simulink model "processor_ks"  (R2025a)
settings: Solver=VariableStepAuto  StartTime=0.0  StopTime=10.0  RelTol=1e-3
(part 1 of 2)
settings Model: Creator=Krutyanjay  LastModifiedBy=Krutyanjay

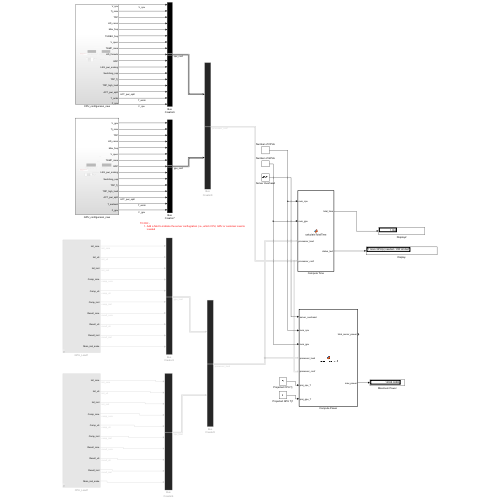
[thumbnail: Simulink's stored preview of the top-level diagram]
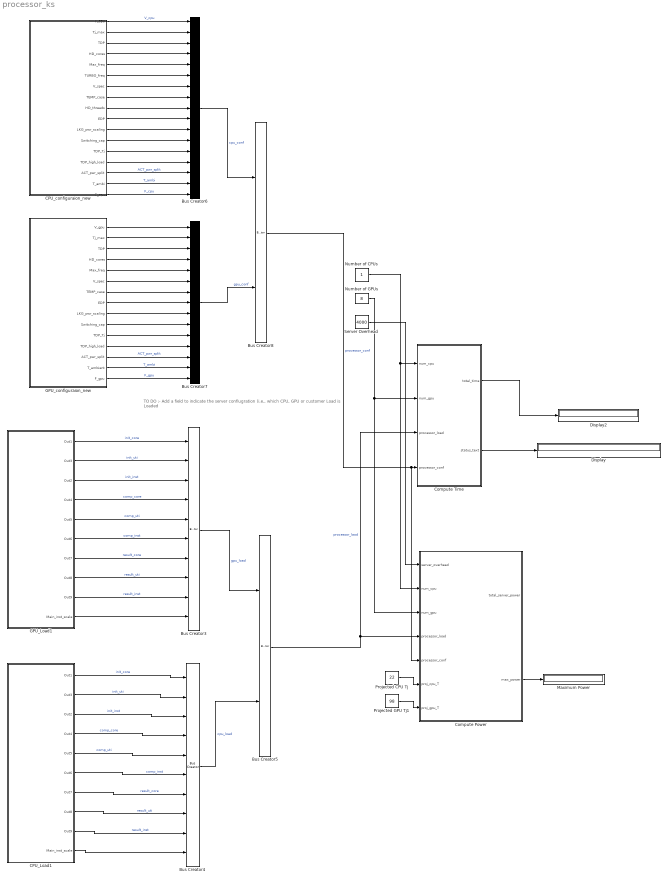
== system processor_ks ==
  note: TO DO :-
      | Add a field to indicate the server confiugration (i.e., which CPU, GPU or customer Load is Loaded
  Bus Creator3 : BusCreator  Inputs=10  OutDataTypeStr=Bus: gpu_load
  Bus Creator4 : BusCreator  Inputs=10  OutDataTypeStr=Bus: cpu_load
  Bus Creator5 : BusCreator  Inputs=2  OutDataTypeStr=Bus: processor_load
  Bus Creator6 : BusCreator  Inputs=17  OutDataTypeStr=Bus: cpu_conf
  Bus Creator7 : BusCreator  Inputs=15  OutDataTypeStr=Bus: gpu_conf
  Bus Creator8 : BusCreator  Inputs=2  OutDataTypeStr=Bus: processor_conf
  CPU_Load1 : Subsystem  mask{Init_core=30, Init_uti=0.5, Init_inst=500000, Comp_core=0, Comp_uti=0, Comp_inst=0, Result_core=20, Result_uti=0.5, Result_inst=100000, Main_inst_scale=1}
      mask prompts: Init_core "Initilization Phase cores"; Init_uti "Total initilization core utilization"; Init_inst "Number of instructions for initilization"; Comp_core "Compute Phase cores"; Comp_uti "Total Compute core utilization"; Comp_inst "Number of isntrutction for compute"; Result_core "Result Phase cores"; Result_uti "Total result core utilization"; Result_inst "Number of instructions for result"; Main_inst_scale "Main Phase Instruction scaling"
      mask DialogControl saveButton Prompt: Save to CSV
      mask DialogControl loadButton Prompt: Load from CSV
  CPU_configuraion_new : Subsystem
  Compute Power : MATLAB Function  TreatAsAtomicUnit=on
  Compute Time : MATLAB Function  TreatAsAtomicUnit=on
  Display : Display
  Display2 : Display
  GPU_Load1 : Subsystem  mask{Init_core=12, Init_uti=0.1, Init_inst=40000, Comp_core=250000, Comp_uti=0.75, Comp_inst=1000000000000000, Result_core=5, Result_uti=0.1, Result_inst=10000, Main_inst_scale=2.8}
      mask prompts: Init_core "Initilization Phase cores"; Init_uti "Total initilization core utilization"; Init_inst "Number of instructions for initilization"; Comp_core "Compute Phase cores"; Comp_uti "Total Compute core utilization"; Comp_inst "Number of isntrutction for compute"; Result_core "Result Phase cores"; Result_uti "Total result core utilization"; Result_inst "Number of instructions for result"; Main_inst_scale "Main Phase Instruction Scaling"
      mask DialogControl saveButton Prompt: Save to CSV
      mask DialogControl loadButton Prompt: Load from CSV
  GPU_configuraion_new : Subsystem
  Maximum Power : Display
  Number of CPUs : Constant
  Number of GPUs : Constant  Value=8
  Projected CPU Tj : Constant  Value=22
  Projected GPU Tj1 : Constant  Value=98
  Server Overhead : Constant  Value=4000
  wires:
  GPU_Load1/7(Out7) -> Bus Creator3/7  "result_core"
  CPU_Load1/5(Out5) -> Bus Creator4/5  "comp_uti"
  GPU_Load1/2(Out3) -> Bus Creator3/2  "init_uti"
  GPU_Load1/3(Out2) -> Bus Creator3/3  "init_inst"
  CPU_Load1/8(Out8) -> Bus Creator4/8  "result_uti"
  CPU_Load1/1(Out1) -> Bus Creator4/1  "init_core"
  CPU_Load1/3(Out2) -> Bus Creator4/3  "init_inst"
  GPU_Load1/6(Out6) -> Bus Creator3/6  "comp_inst"
  GPU_Load1/1(Out1) -> Bus Creator3/1  "init_core"
  CPU_Load1/4(Out4) -> Bus Creator4/4  "comp_core"
  GPU_Load1/4(Out4) -> Bus Creator3/4  "comp_core"
  GPU_Load1/9(Out9) -> Bus Creator3/9  "result_inst"
  CPU_Load1/2(Out3) -> Bus Creator4/2  "init_uti"
  CPU_Load1/9(Out9) -> Bus Creator4/9  "result_inst"
  GPU_Load1/8(Out8) -> Bus Creator3/8  "result_uti"
  CPU_Load1/6(Out6) -> Bus Creator4/6  "comp_inst"
  GPU_Load1/5(Out5) -> Bus Creator3/5  "comp_uti"
  CPU_Load1/7(Out7) -> Bus Creator4/7  "result_core"
  Bus Creator6/1 -> Bus Creator8/1  "cpu_conf"
  Bus Creator7/1 -> Bus Creator8/2  "gpu_conf"
  Bus Creator8/1 -> Compute Power/5(processor_conf), Compute Time/4(processor_conf)  "processor_conf"
  Bus Creator5/1 -> Compute Time/3(processor_load), Compute Power/4(processor_load)  "processor_laod"
  Compute Time/1(total_time) -> Display2/1
  Number of CPUs/1 -> Compute Time/1(num_cpu), Compute Power/2(num_cpu)
  Number of GPUs/1 -> Compute Power/3(num_gpu), Compute Time/2(num_gpu)
  Server Overhead/1 -> Compute Power/1(server_overhead)
  Compute Power/2(max_power) -> Maximum Power/1
  Compute Time/2(status_text) -> Display/1
  GPU_configuraion_new/1(V_gpu) -> Bus Creator7/1
  GPU_configuraion_new/2(Tj_max) -> Bus Creator7/2
  GPU_configuraion_new/3(TDP) -> Bus Creator7/3
  GPU_configuraion_new/4(HD_cores) -> Bus Creator7/4
  GPU_configuraion_new/5(Max_freq) -> Bus Creator7/5
  GPU_configuraion_new/6(V_spec) -> Bus Creator7/6
  GPU_configuraion_new/7(TEMP_case) -> Bus Creator7/7
  GPU_configuraion_new/8(EDP) -> Bus Creator7/8
  GPU_configuraion_new/9(LKG_pwr_scaling) -> Bus Creator7/9
  GPU_configuraion_new/10(Switching_cap) -> Bus Creator7/10
  GPU_configuraion_new/11(TDP_Tj) -> Bus Creator7/11
  GPU_configuraion_new/12(TDP_high_load) -> Bus Creator7/12
  GPU_configuraion_new/13(ACT_pwr_split) -> Bus Creator7/13  "ACT_pwr_split"
  CPU_configuraion_new/1(V_cpu) -> Bus Creator6/1  "V_cpu"
  CPU_configuraion_new/2(Tj_max) -> Bus Creator6/2
  CPU_configuraion_new/3(TDP) -> Bus Creator6/3
  CPU_configuraion_new/4(HD_cores) -> Bus Creator6/4
  CPU_configuraion_new/5(Max_freq) -> Bus Creator6/5
  CPU_configuraion_new/6(TURBO_freq) -> Bus Creator6/6
  CPU_configuraion_new/7(V_spec) -> Bus Creator6/7
  CPU_configuraion_new/8(TEMP_case) -> Bus Creator6/8
  CPU_configuraion_new/9(HD_threads) -> Bus Creator6/9
  CPU_configuraion_new/10(EDP) -> Bus Creator6/10
  CPU_configuraion_new/11(LKG_pwr_scaling) -> Bus Creator6/11
  CPU_configuraion_new/12(Switching_cap) -> Bus Creator6/12
  CPU_configuraion_new/13(TDP_Tj) -> Bus Creator6/13
  CPU_configuraion_new/14(TDP_high_load) -> Bus Creator6/14
  CPU_configuraion_new/15(ACT_pwr_split) -> Bus Creator6/15  "ACT_pwr_split"
  Bus Creator3/1 -> Bus Creator5/1  "gpu_load"
  Bus Creator4/1 -> Bus Creator5/2  "cpu_load"
  CPU_configuraion_new/16(T_ambi) -> Bus Creator6/16  "T_ambi"
  GPU_configuraion_new/14(T_ambient) -> Bus Creator7/14  "T_ambi"
  CPU_configuraion_new/17(F_cpu) -> Bus Creator6/17  "F_cpu"
  GPU_configuraion_new/15(F_gpu) -> Bus Creator7/15  "F_gpu"
  GPU_Load1/10(Main_inst_scale) -> Bus Creator3/10
  CPU_Load1/10(Main_inst_scale) -> Bus Creator4/10
  Projected CPU Tj/1 -> Compute Power/6(proj_cpu_T)
  Projected GPU Tj1/1 -> Compute Power/7(proj_gpu_T)

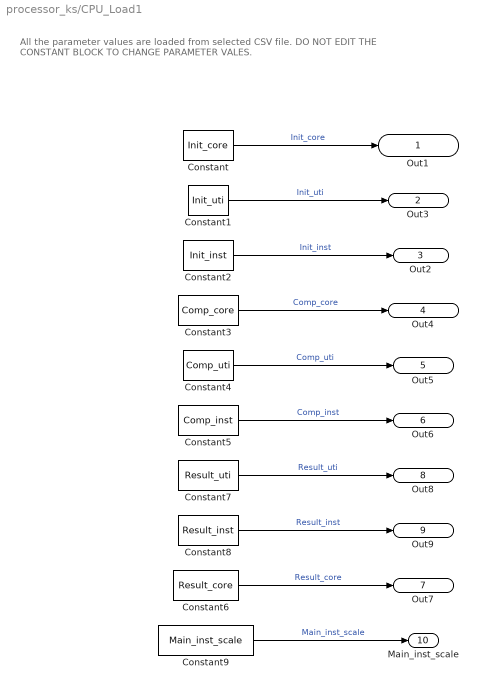
== system processor_ks/CPU_Load1 ==
  note: All the parameter values are loaded from selected CSV file.
      | DO NOT EDIT THE CONSTANT BLOCK TO CHANGE PARAMETER VALES.
  Constant : Constant  Value=Init_core
  Constant1 : Constant  Value=Init_uti
  Constant2 : Constant  Value=Init_inst
  Constant3 : Constant  Value=Comp_core
  Constant4 : Constant  Value=Comp_uti
  Constant5 : Constant  Value=Comp_inst
  Constant6 : Constant  Value=Result_core
  Constant7 : Constant  Value=Result_uti
  Constant8 : Constant  Value=Result_inst
  Constant9 : Constant  Value=Main_inst_scale
  Out1 : Outport
  Out3 : Outport  Port=2
  Out2 : Outport  Port=3
  Out4 : Outport  Port=4
  Out5 : Outport  Port=5
  Out6 : Outport  Port=6
  Out7 : Outport  Port=7
  Out8 : Outport  Port=8
  Out9 : Outport  Port=9
  Main_inst_scale : Outport  Port=10
  wires:
  Constant7/1 -> Out8/1  "Result_uti"
  Constant5/1 -> Out6/1  "Comp_inst"
  Constant3/1 -> Out4/1  "Comp_core"
  Constant1/1 -> Out3/1  "Init_uti"
  Constant4/1 -> Out5/1  "Comp_uti"
  Constant6/1 -> Out7/1  "Result_core"
  Constant/1 -> Out1/1  "Init_core"
  Constant2/1 -> Out2/1  "Init_inst"
  Constant8/1 -> Out9/1  "Result_inst"
  Constant9/1 -> Main_inst_scale/1  "Main_inst_scale"

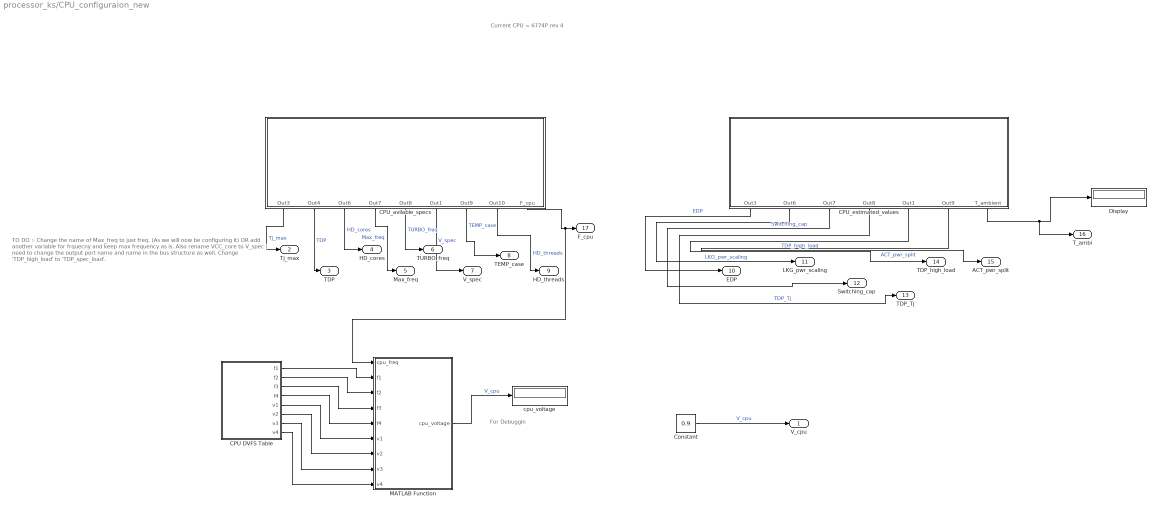
== system processor_ks/CPU_configuraion_new ==
  note: TO DO :-
      | Change the name of Max_freq to just freq. (As we will now be configuring it)
      | OR add another variable for frquecny and keep max frequency as is.
      | Also rename VCC_core to V_spec ( need to change the output port name and name in the bus structure as well.
      | Change 'TDP_high_load' to 'TDP_spec_load'.
  note: For Debuggin
  note: Current CPU = 6774P rev 4
  CPU DVFS Table : Subsystem  mask{F1=2.5e9, F2=2.3e9, F3=1.8e9, F4=1.4e9, V1=1.5, V2=1.3, V3=1.1, V4=0.9, loaded_device_name=hello}
      mask prompts: loaded_device_name "Device DVFS"
      mask DialogControl save_dvfs_button Prompt: Save To CSV
      mask DialogControl load_dvfs_button Prompt: Load From CSV
  CPU_avilable_specs : Subsystem  mask{TURBO_freq=3.9e9, V_spec=1.5, TEMP_case=85, Tj_max=100, HD_cores=40, Max_freq=2500000000, TDP=235, HD_threads=128, F_cpu=1.4e9}
      mask DialogControl save_button Prompt: Save To CSV
      mask DialogControl load_button Prompt: Load From CSV
  CPU_estimated_values : Subsystem  mask{EDP=587.5, LKG_pwr_scaling=394.5, Switching_cap=28.35, TDP_Tj=70, TDP_high_load=0.7, ACT_pwr_split=0.5, T_ambient=20}
      mask DialogControl save_button Prompt: Save To CSV
      mask DialogControl load_button Prompt: Load From CSV
  Constant : Constant  Value=0.9
  Display : Display
  MATLAB Function : MATLAB Function  TreatAsAtomicUnit=on
  cpu_voltage : Display
  V_cpu : Outport
  Tj_max : Outport  Port=2
  TDP : Outport  Port=3
  HD_cores : Outport  Port=4
  Max_freq : Outport  Port=5
  TURBO_freq : Outport  Port=6
  V_spec : Outport  Port=7
  TEMP_case : Outport  Port=8
  HD_threads : Outport  Port=9
  EDP : Outport  Port=10
  LKG_pwr_scaling : Outport  Port=11
  Switching_cap : Outport  Port=12
  TDP_Tj : Outport  Port=13
  TDP_high_load : Outport  Port=14
  ACT_pwr_split : Outport  Port=15
  T_ambi : Outport  Port=16
  F_cpu : Outport  Port=17
  wires:
  CPU_avilable_specs/1(Out3) -> Tj_max/1  "Tj_max"
  CPU_avilable_specs/2(Out4) -> TDP/1  "TDP"
  CPU_avilable_specs/3(Out6) -> HD_cores/1  "HD_cores"
  CPU_avilable_specs/4(Out7) -> Max_freq/1  "Max_freq"
  CPU_avilable_specs/5(Out8) -> TURBO_freq/1  "TURBO_freq"
  CPU_avilable_specs/7(Out9) -> TEMP_case/1  "TEMP_case"
  CPU_avilable_specs/8(Out10) -> HD_threads/1  "HD_threads"
  CPU_estimated_values/1(Out3) -> EDP/1  "EDP"
  CPU_estimated_values/2(Out6) -> LKG_pwr_scaling/1  "LKG_pwr_scaling"
  CPU_estimated_values/3(Out7) -> Switching_cap/1  "Switching_cap"
  CPU_estimated_values/4(Out8) -> TDP_Tj/1  "TDP_Tj"
  CPU_estimated_values/5(Out1) -> TDP_high_load/1  "TDP_high_load"
  CPU_estimated_values/6(Out9) -> ACT_pwr_split/1  "ACT_pwr_split"
  CPU DVFS Table/1(f1) -> MATLAB Function/2(f1)
  CPU DVFS Table/2(f2) -> MATLAB Function/3(f2)
  CPU DVFS Table/3(f3) -> MATLAB Function/4(f3)
  CPU DVFS Table/4(f4) -> MATLAB Function/5(f4)
  CPU DVFS Table/5(v1) -> MATLAB Function/6(v1)
  CPU DVFS Table/6(v2) -> MATLAB Function/7(v2)
  CPU DVFS Table/7(v3) -> MATLAB Function/8(v3)
  CPU DVFS Table/8(v4) -> MATLAB Function/9(v4)
  MATLAB Function/1(cpu_voltage) -> cpu_voltage/1  "V_cpu"
  CPU_avilable_specs/6(Out1) -> V_spec/1  "V_spec"
  CPU_estimated_values/7(T_ambient) -> T_ambi/1, Display/1
  CPU_avilable_specs/9(F_cpu) -> MATLAB Function/1(cpu_freq), F_cpu/1
  Constant/1 -> V_cpu/1  "V_cpu"

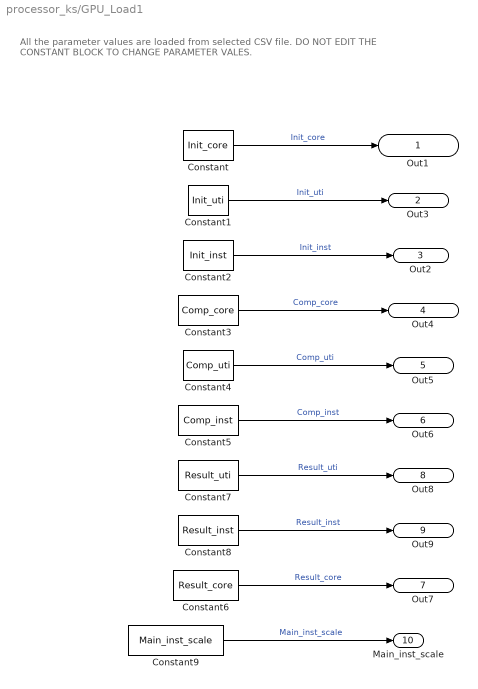
== system processor_ks/GPU_Load1 ==
  note: All the parameter values are loaded from selected CSV file.
      | DO NOT EDIT THE CONSTANT BLOCK TO CHANGE PARAMETER VALES.
  Constant : Constant  Value=Init_core
  Constant1 : Constant  Value=Init_uti
  Constant2 : Constant  Value=Init_inst
  Constant3 : Constant  Value=Comp_core
  Constant4 : Constant  Value=Comp_uti
  Constant5 : Constant  Value=Comp_inst
  Constant6 : Constant  Value=Result_core
  Constant7 : Constant  Value=Result_uti
  Constant8 : Constant  Value=Result_inst
  Constant9 : Constant  Value=Main_inst_scale
  Out1 : Outport
  Out3 : Outport  Port=2
  Out2 : Outport  Port=3
  Out4 : Outport  Port=4
  Out5 : Outport  Port=5
  Out6 : Outport  Port=6
  Out7 : Outport  Port=7
  Out8 : Outport  Port=8
  Out9 : Outport  Port=9
  Main_inst_scale : Outport  Port=10
  wires:
  Constant7/1 -> Out8/1  "Result_uti"
  Constant5/1 -> Out6/1  "Comp_inst"
  Constant3/1 -> Out4/1  "Comp_core"
  Constant1/1 -> Out3/1  "Init_uti"
  Constant4/1 -> Out5/1  "Comp_uti"
  Constant6/1 -> Out7/1  "Result_core"
  Constant/1 -> Out1/1  "Init_core"
  Constant2/1 -> Out2/1  "Init_inst"
  Constant8/1 -> Out9/1  "Result_inst"
  Constant9/1 -> Main_inst_scale/1  "Main_inst_scale"

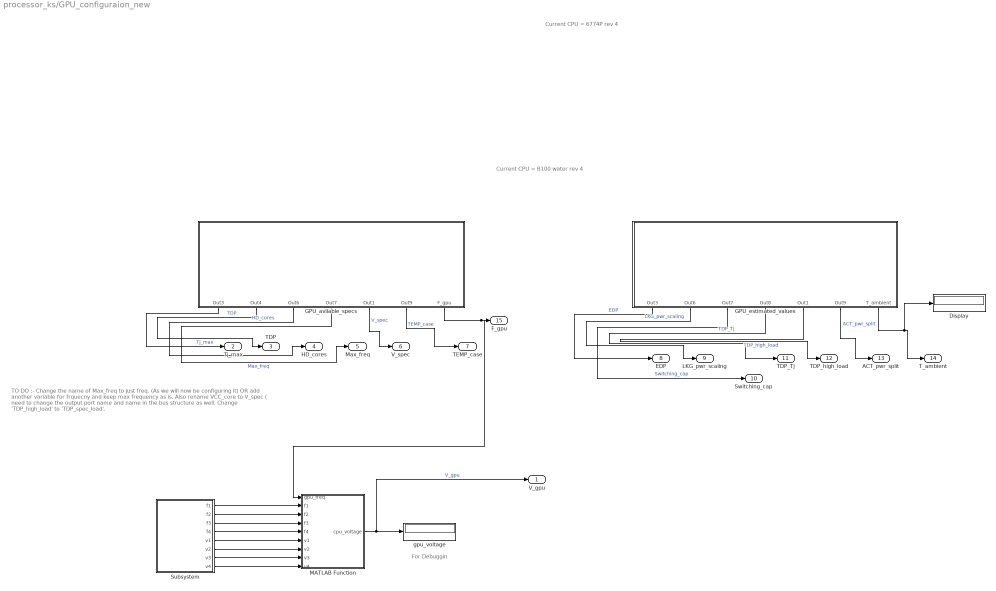
== system processor_ks/GPU_configuraion_new ==
  note: For Debuggin
  note: TO DO :-
      | Change the name of Max_freq to just freq. (As we will now be configuring it)
      | OR add another variable for frquecny and keep max frequency as is.
      | Also rename VCC_core to V_spec ( need to change the output port name and name in the bus structure as well.
      | Change 'TDP_high_load' to 'TDP_spec_load'.
  note: Current CPU = 6774P rev 4
  note: Current CPU = B100 water rev 4
  Display : Display
  GPU_avilable_specs : Subsystem  mask{V_spec=1, TEMP_case=85, Tj_max=95, HD_cores=30000, Max_freq=1900000000, TDP=1400, F_gpu=1.4e9}
      mask DialogControl save_button Prompt: Save To CSV
      mask DialogControl load_button Prompt: Load From CSV
  GPU_estimated_values : Subsystem  mask{EDP=2286.7, LKG_pwr_scaling=1, Switching_cap=368.42, TDP_Tj=70, TDP_high_load=0.75, ACT_pwr_split=0.5, T_ambient=20}
      mask DialogControl save_button Prompt: Save To CSV
      mask DialogControl load_button Prompt: Load From CSV
  MATLAB Function : MATLAB Function  TreatAsAtomicUnit=on
  Subsystem : Subsystem  mask{F1=1.9e9, F2=1.7e9, F3=1.4e9, F4=1.3e9, V1=1, V2=0.8, V3=0.7, V4=0.5, loaded_device_name=0}
      mask prompts: loaded_device_name "Device's DVFS"
      mask DialogControl save_dvfs_button Prompt: Save To CSV
      mask DialogControl load_dvfs_button Prompt: Load from CSV
  gpu_voltage : Display
  V_gpu : Outport
  Tj_max : Outport  Port=2
  TDP : Outport  Port=3
  HD_cores : Outport  Port=4
  Max_freq : Outport  Port=5
  V_spec : Outport  Port=6
  TEMP_case : Outport  Port=7
  EDP : Outport  Port=8
  LKG_pwr_scaling : Outport  Port=9
  Switching_cap : Outport  Port=10
  TDP_Tj : Outport  Port=11
  TDP_high_load : Outport  Port=12
  ACT_pwr_split : Outport  Port=13
  T_ambient : Outport  Port=14
  F_gpu : Outport  Port=15
  wires:
  GPU_avilable_specs/1(Out3) -> Tj_max/1  "Tj_max"
  GPU_avilable_specs/2(Out4) -> TDP/1  "TDP"
  GPU_avilable_specs/3(Out6) -> HD_cores/1  "HD_cores"
  GPU_avilable_specs/4(Out7) -> Max_freq/1  "Max_freq"
  GPU_avilable_specs/5(Out1) -> V_spec/1  "V_spec"
  GPU_avilable_specs/6(Out9) -> TEMP_case/1  "TEMP_case"
  GPU_estimated_values/1(Out3) -> EDP/1  "EDP"
  GPU_estimated_values/2(Out6) -> LKG_pwr_scaling/1  "LKG_pwr_scaling"
  GPU_estimated_values/3(Out7) -> Switching_cap/1  "Switching_cap"
  GPU_estimated_values/4(Out8) -> TDP_Tj/1  "TDP_Tj"
  GPU_estimated_values/5(Out1) -> TDP_high_load/1  "TDP_high_load"
  GPU_estimated_values/6(Out9) -> ACT_pwr_split/1  "ACT_pwr_split"
  MATLAB Function/1(cpu_voltage) -> V_gpu/1, gpu_voltage/1  "V_gpu"
  Subsystem/3(f3) -> MATLAB Function/4(f3)
  Subsystem/2(f2) -> MATLAB Function/3(f2)
  Subsystem/6(v2) -> MATLAB Function/7(v2)
  Subsystem/8(v4) -> MATLAB Function/9(v4)
  Subsystem/7(v3) -> MATLAB Function/8(v3)
  Subsystem/1(f1) -> MATLAB Function/2(f1)
  Subsystem/4(f4) -> MATLAB Function/5(f4)
  Subsystem/5(v1) -> MATLAB Function/6(v1)
  GPU_estimated_values/7(T_ambient) -> Display/1, T_ambient/1
  GPU_avilable_specs/7(F_gpu) -> MATLAB Function/1(gpu_freq), F_gpu/1

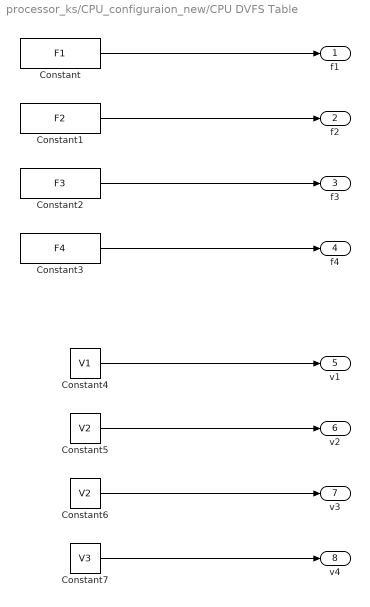
== system processor_ks/CPU_configuraion_new/CPU DVFS Table ==
  Constant : Constant  Value=F1
  Constant1 : Constant  Value=F2
  Constant2 : Constant  Value=F3
  Constant3 : Constant  Value=F4
  Constant4 : Constant  Value=V1
  Constant5 : Constant  Value=V2
  Constant6 : Constant  Value=V2
  Constant7 : Constant  Value=V3
  f1 : Outport
  f2 : Outport  Port=2
  f3 : Outport  Port=3
  f4 : Outport  Port=4
  v1 : Outport  Port=5
  v2 : Outport  Port=6
  v3 : Outport  Port=7
  v4 : Outport  Port=8
  wires:
  Constant/1 -> f1/1
  Constant1/1 -> f2/1
  Constant2/1 -> f3/1
  Constant3/1 -> f4/1
  Constant7/1 -> v4/1
  Constant6/1 -> v3/1
  Constant5/1 -> v2/1
  Constant4/1 -> v1/1

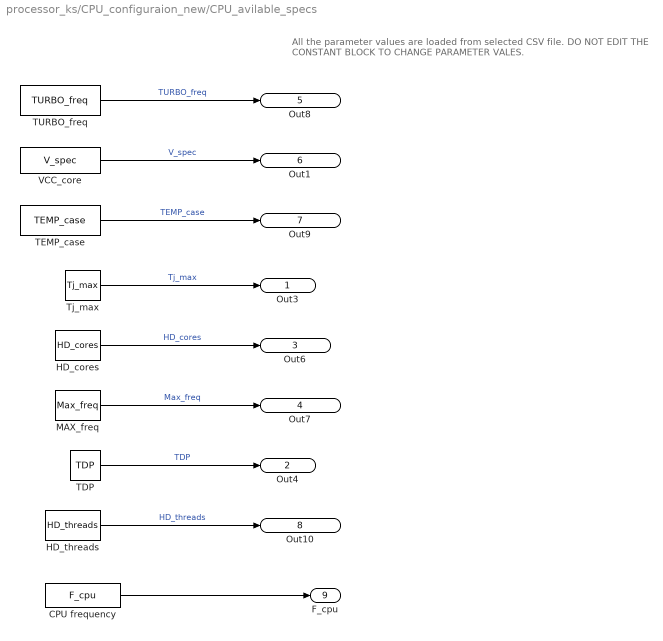
== system processor_ks/CPU_configuraion_new/CPU_avilable_specs ==
  note: All the parameter values are loaded from selected CSV file.
      | DO NOT EDIT THE CONSTANT BLOCK TO CHANGE PARAMETER VALES.
  CPU frequency : Constant  Value=F_cpu
  HD_cores : Constant  Value=HD_cores
  HD_threads : Constant  Value=HD_threads
  MAX_freq : Constant  Value=Max_freq
  TDP : Constant  Value=TDP
  TEMP_case : Constant  Value=TEMP_case
  TURBO_freq : Constant  Value=TURBO_freq
  Tj_max : Constant  Value=Tj_max
  VCC_core : Constant  Value=V_spec
  Out3 : Outport
  Out4 : Outport  Port=2
  Out6 : Outport  Port=3
  Out7 : Outport  Port=4
  Out8 : Outport  Port=5
  Out1 : Outport  Port=6
  Out9 : Outport  Port=7
  Out10 : Outport  Port=8
  F_cpu : Outport  Port=9
  wires:
  HD_threads/1 -> Out10/1  "HD_threads"
  TDP/1 -> Out4/1  "TDP"
  MAX_freq/1 -> Out7/1  "Max_freq"
  HD_cores/1 -> Out6/1  "HD_cores"
  Tj_max/1 -> Out3/1  "Tj_max"
  TEMP_case/1 -> Out9/1  "TEMP_case"
  TURBO_freq/1 -> Out8/1  "TURBO_freq"
  VCC_core/1 -> Out1/1  "V_spec"
  CPU frequency/1 -> F_cpu/1

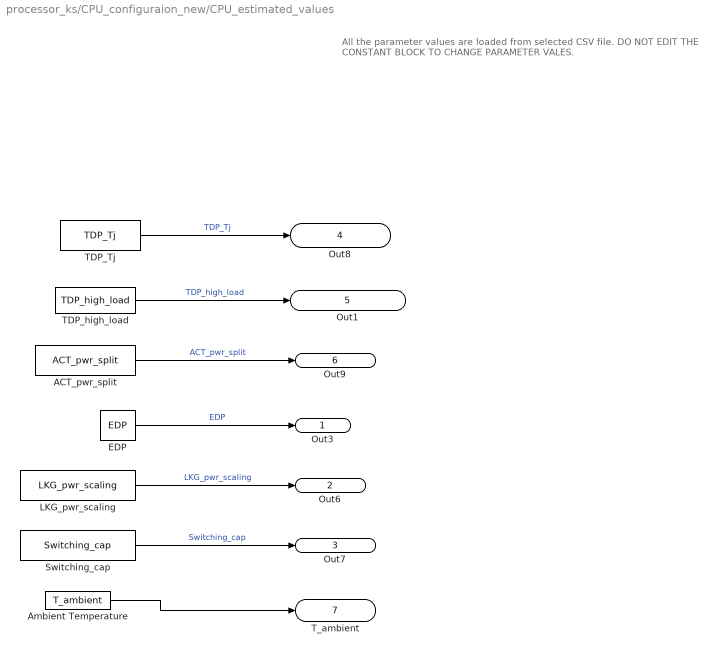
== system processor_ks/CPU_configuraion_new/CPU_estimated_values ==
  note: All the parameter values are loaded from selected CSV file.
      | DO NOT EDIT THE CONSTANT BLOCK TO CHANGE PARAMETER VALES.
  ACT_pwr_split : Constant  Value=ACT_pwr_split
  Ambient Temperature : Constant  Value=T_ambient
  EDP : Constant  Value=EDP
  LKG_pwr_scaling : Constant  Value=LKG_pwr_scaling
  Switching_cap : Constant  Value=Switching_cap
  TDP_Tj : Constant  Value=TDP_Tj
  TDP_high_load : Constant  Value=TDP_high_load
  Out3 : Outport
  Out6 : Outport  Port=2
  Out7 : Outport  Port=3
  Out8 : Outport  Port=4
  Out1 : Outport  Port=5
  Out9 : Outport  Port=6
  T_ambient : Outport  Port=7
  wires:
  Switching_cap/1 -> Out7/1  "Switching_cap"
  LKG_pwr_scaling/1 -> Out6/1  "LKG_pwr_scaling"
  EDP/1 -> Out3/1  "EDP"
  ACT_pwr_split/1 -> Out9/1  "ACT_pwr_split"
  TDP_Tj/1 -> Out8/1  "TDP_Tj"
  TDP_high_load/1 -> Out1/1  "TDP_high_load"
  Ambient Temperature/1 -> T_ambient/1

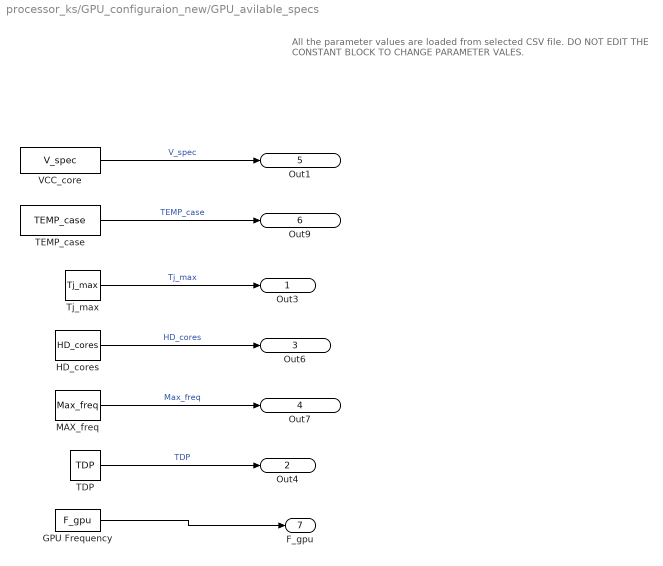
== system processor_ks/GPU_configuraion_new/GPU_avilable_specs ==
  note: All the parameter values are loaded from selected CSV file.
      | DO NOT EDIT THE CONSTANT BLOCK TO CHANGE PARAMETER VALES.
  GPU Frequency : Constant  Value=F_gpu
  HD_cores : Constant  Value=HD_cores
  MAX_freq : Constant  Value=Max_freq
  TDP : Constant  Value=TDP
  TEMP_case : Constant  Value=TEMP_case
  Tj_max : Constant  Value=Tj_max
  VCC_core : Constant  Value=V_spec
  Out3 : Outport
  Out4 : Outport  Port=2
  Out6 : Outport  Port=3
  Out7 : Outport  Port=4
  Out1 : Outport  Port=5
  Out9 : Outport  Port=6
  F_gpu : Outport  Port=7
  wires:
  TDP/1 -> Out4/1  "TDP"
  MAX_freq/1 -> Out7/1  "Max_freq"
  HD_cores/1 -> Out6/1  "HD_cores"
  Tj_max/1 -> Out3/1  "Tj_max"
  TEMP_case/1 -> Out9/1  "TEMP_case"
  VCC_core/1 -> Out1/1  "V_spec"
  GPU Frequency/1 -> F_gpu/1

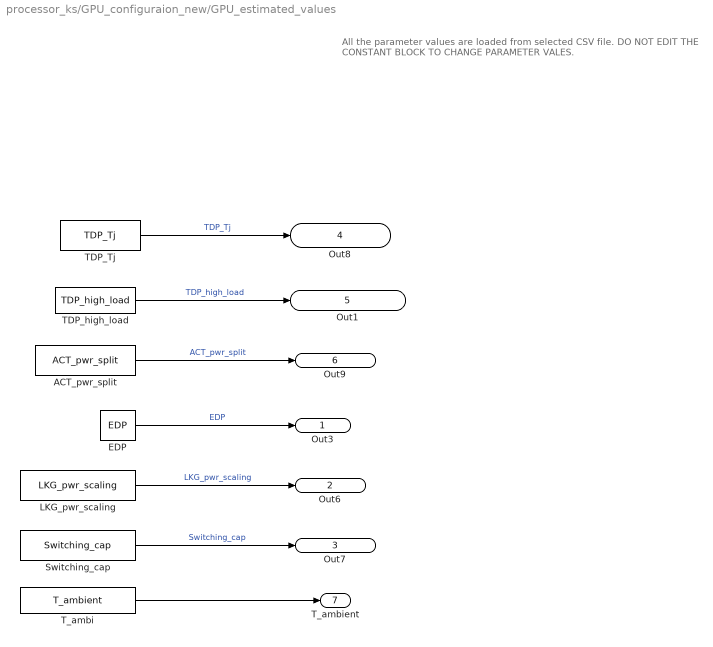
== system processor_ks/GPU_configuraion_new/GPU_estimated_values ==
  note: All the parameter values are loaded from selected CSV file.
      | DO NOT EDIT THE CONSTANT BLOCK TO CHANGE PARAMETER VALES.
  ACT_pwr_split : Constant  Value=ACT_pwr_split
  EDP : Constant  Value=EDP
  LKG_pwr_scaling : Constant  Value=LKG_pwr_scaling
  Switching_cap : Constant  Value=Switching_cap
  TDP_Tj : Constant  Value=TDP_Tj
  TDP_high_load : Constant  Value=TDP_high_load
  T_ambi : Constant  Value=T_ambient
  Out3 : Outport
  Out6 : Outport  Port=2
  Out7 : Outport  Port=3
  Out8 : Outport  Port=4
  Out1 : Outport  Port=5
  Out9 : Outport  Port=6
  T_ambient : Outport  Port=7
  wires:
  Switching_cap/1 -> Out7/1  "Switching_cap"
  LKG_pwr_scaling/1 -> Out6/1  "LKG_pwr_scaling"
  EDP/1 -> Out3/1  "EDP"
  ACT_pwr_split/1 -> Out9/1  "ACT_pwr_split"
  TDP_Tj/1 -> Out8/1  "TDP_Tj"
  TDP_high_load/1 -> Out1/1  "TDP_high_load"
  T_ambi/1 -> T_ambient/1

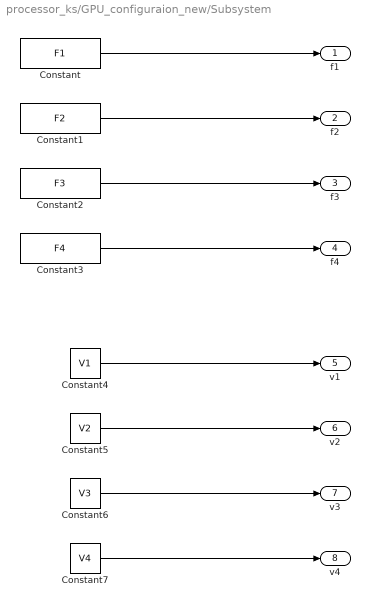
== system processor_ks/GPU_configuraion_new/Subsystem ==
  Constant : Constant  Value=F1
  Constant1 : Constant  Value=F2
  Constant2 : Constant  Value=F3
  Constant3 : Constant  Value=F4
  Constant4 : Constant  Value=V1
  Constant5 : Constant  Value=V2
  Constant6 : Constant  Value=V3
  Constant7 : Constant  Value=V4
  f1 : Outport
  f2 : Outport  Port=2
  f3 : Outport  Port=3
  f4 : Outport  Port=4
  v1 : Outport  Port=5
  v2 : Outport  Port=6
  v3 : Outport  Port=7
  v4 : Outport  Port=8
  wires:
  Constant/1 -> f1/1
  Constant1/1 -> f2/1
  Constant2/1 -> f3/1
  Constant3/1 -> f4/1
  Constant7/1 -> v4/1
  Constant6/1 -> v3/1
  Constant5/1 -> v2/1
  Constant4/1 -> v1/1

== matlab function processor_ks/GPU_configuraion_new/MATLAB Function ==
  data: gpu_freq input; f1 input; f2 input; f3 input; f4 input; v1 input; v2 input; v3 input; v4 input; cpu_voltage output
function cpu_voltage = fcn(gpu_freq, f1, f2, f3, f4, v1, v2, v3, v4)
%#codegen
% This function performs a DVFS lookup based on the provided tables.
% It takes a 'gpu_freq' and a set of F-V pairs (f1,v1), (f2,v2), etc.
% and returns the corresponding voltage.

%% 1. Build the DVFS tables (arrays)
% Combine the separate scalar inputs into two vectors (arrays) that
% the interp1 function can use for the lookup.

freq_table = [f1, f2, f3, f4];
volt_table = [v1, v2, v3, v4];

%% 2. Perform the Lookup
% Use 1D interpolation to find the voltage that matches the gpu_freq.
%
% 'nearest' - This snaps to the closest frequency in your table. 
% 'extrap'  - If gpu_freq is outside the table's range (higher or
%             lower), this will use the nearest end value (e.g., v1 or v4)
%             instead of returning an error (NaN).

cpu_voltage = interp1(freq_table, volt_table, gpu_freq, 'nearest', 'extrap');

end

== matlab function processor_ks/CPU_configuraion_new/MATLAB Function ==
  data: cpu_freq input; f1 input; f2 input; f3 input; f4 input; v1 input; v2 input; v3 input; v4 input; cpu_voltage output
function cpu_voltage = fcn(cpu_freq, f1, f2, f3, f4, v1, v2, v3, v4)
%#codegen
% This function performs a DVFS lookup based on the provided tables.
% It takes a 'cpu_freq' and a set of F-V pairs (f1,v1), (f2,v2), etc.
% and returns the corresponding voltage.

%% 1. Build the DVFS tables (arrays)
% Combine the separate scalar inputs into two vectors (arrays) that
% the interp1 function can use for the lookup.

freq_table = [f1, f2, f3, f4];
volt_table = [v1, v2, v3, v4];

%% 2. Perform the Lookup
% Use 1D interpolation to find the voltage that matches the cpu_freq.
%
% 'nearest' - This snaps to the closest frequency in your table. This
%             is the correct method for a discrete DVFS table.
% 'extrap'  - If cpu_freq is outside the table's range (higher or
%             lower), this will use the nearest end value (e.g., v1 or v4)
%             instead of returning an error (NaN).

cpu_voltage = interp1(freq_table, volt_table, cpu_freq, 'nearest', 'extrap');

end

== matlab function processor_ks/Compute Time ==
  data: num_cpu input; num_gpu input; processor_load input; processor_conf input; total_time output; status_text output
function [total_time,status_text] = calculateTotalTime(num_cpu, num_gpu, processor_load, processor_conf)
    % This function calculates the total processing time for a server
    % based on the number of CPUs/GPUs and the given workload.
    % NOTE :- This funstion works on the assumstion that every instruction
    % is completed in a single clock cycle.

    %% --- 1. Calculate Total Server Hardware ---
    % The 'processor_conf' struct holds the specs for a SINGLE device.
    % We multiply by the number of devices to get the total server resources.

    % --- Output Initialization ---
    % We MUST assign default values to all outputs at the top.
    total_time = 0;
    status_text = "Calculating..."; % Assign a default string

    % Multi Precision scaling Factor
    Multi_inst_cpu_scale = processor_load.cpu_load.Main_inst_scale;
    Multi_inst_gpu_scale = processor_load.gpu_load.Main_inst_scale;

    % --- Total CPU Resources ---
    single_cpu_cores = processor_conf.cpu_conf.HD_cores;
    total_cpu_cores = num_cpu * single_cpu_cores;
    % techinically its per core frequency
    cpu_freq = processor_conf.cpu_conf.F_cpu;

    % --- Total GPU Resources ---
    single_gpu_cores = processor_conf.gpu_conf.HD_cores;
    total_gpu_cores = num_gpu * single_gpu_cores;
    gpu_freq  = processor_conf.gpu_conf.F_gpu;
    % ----- Software load parameters -----------------
    % Number of parallel instructions the CPU kernel can divide the given load into
    SD_cores_cpu_init = processor_load.cpu_load.init_core;
    SD_cores_cpu_main = processor_load.cpu_load.comp_core;
    SD_cores_cpu_result = processor_load.cpu_load.result_core;
    SD_cores_gpu_init = processor_load.gpu_load.init_core;
    SD_cores_gpu_main = processor_load.gpu_load.comp_core;
    SD_cores_gpu_result = processor_load.gpu_load.result_core;
    % print parameters used ( Debugging and sanity check)
    % fprintf('------------ TIME === Sanity check start === -------------\n');
    % fprintf('1. CPU and GPU parameters\n');
    % fprintf('Single CPU cores = %f\n',single_cpu_cores);
    % fprintf('Single GPU cores = %f\n',single_gpu_cores);
    % fprintf('Number of CPUs = %f\n',num_cpu);
    % fprintf('Number of GPUs = %f\n',num_gpu);
    % fprintf('CPU core frequency = %f\n',cpu_freq);
    % fprintf('GPU core frequency = %f\n',gpu_freq);
    % fprintf('--------------------------------\n');
    % fprintf('CPU init softwares cores = %f\n',SD_cores_cpu_init);
    % fprintf('CPU main softwares cores = %f\n',SD_cores_cpu_main);
    % fprintf('CPU main Instruction Scaling Factor = %f\n',Multi_inst_cpu_scale);
    % fprintf('CPU result softwares cores = %f\n',SD_cores_cpu_result);
    % fprintf('GPU init softwares cores = %f\n',SD_cores_gpu_init);
    % fprintf('GPU main softwares cores = %f\n',SD_cores_gpu_main);
    % fprintf('GPU main Instruction Scaling Factor = %f\n',Multi_inst_gpu_scale);
    % fprintf('GPU result softwares cores = %f\n',SD_cores_gpu_result);
    % fprintf('--------------------------------\n');

    %% --- A. CPU Time Calculation ---
    % Calculate the "effective" cores (the smaller of software vs. hardware)

    % --- Init Phase ---
    eff_cpu_cores_init = min(SD_cores_cpu_init, total_cpu_cores);
    % check to prevent dividing by 0
    if processor_load.cpu_load.init_inst == 0 || eff_cpu_cores_init == 0 || cpu_freq == 0
        cpu_time_init = 0;
    else
        cpu_time_init = processor_load.cpu_load.init_inst / (eff_cpu_cores_init * cpu_freq );
    end

    % --- Comp / Main Phase ---
    eff_cpu_cores_main = min(SD_cores_cpu_main, total_cpu_cores);
    if processor_load.cpu_load.comp_inst == 0 || eff_cpu_cores_main == 0 || cpu_freq == 0
        cpu_time_main = 0;
    else
        cpu_time_main = processor_load.cpu_load.comp_inst / (eff_cpu_cores_main * cpu_freq * Multi_inst_cpu_scale);
    end

    % --- Result Phase ---
    eff_cpu_cores_result = min(SD_cores_cpu_result, total_cpu_cores);
    if processor_load.cpu_load.result_inst == 0 || eff_cpu_cores_result == 0 || cpu_freq == 0
        cpu_time_result = 0;
    else
        cpu_time_result = processor_load.cpu_load.result_inst / (eff_cpu_cores_result * cpu_freq);
    end

    
    %% --- B. GPU Time Calculation ---
    % Calculate the "effective" cores for the GPU

    % --- Init Phase ---
    eff_gpu_cores_init = min(SD_cores_gpu_init, total_gpu_cores);
    if processor_load.gpu_load.init_inst == 0 || eff_gpu_cores_init == 0 || gpu_freq == 0
        gpu_time_init = 0;
    else
        gpu_time_init = processor_load.gpu_load.init_inst / (eff_gpu_cores_init * gpu_freq);
    end

    % --- Comp / Main Phase ---
    eff_gpu_cores_main = min( SD_cores_gpu_main, total_gpu_cores);
    if processor_load.gpu_load.comp_inst == 0 || eff_gpu_cores_main == 0 || gpu_freq == 0
        gpu_time_main = 0;
    else
        gpu_time_main = processor_load.gpu_load.comp_inst / (eff_gpu_cores_main * gpu_freq * Multi_inst_gpu_scale);
    end

    % --- Result Phase ---
    eff_gpu_cores_result = min(SD_cores_gpu_result, total_gpu_cores);
    if processor_load.gpu_load.result_inst == 0 || eff_gpu_cores_result == 0 || gpu_freq == 0
        gpu_time_result = 0;
    else
        gpu_time_result = processor_load.gpu_load.result_inst / (eff_gpu_cores_result * gpu_freq);
    end

    %% --- C. Combine Parallel Phase Times ---
    % The time for each phase is determined by the slower of the two processors (CPU or GPU).
    time_init   = max(cpu_time_init, gpu_time_init);
    time_main   = max(cpu_time_main, gpu_time_main);
    time_result = max(cpu_time_result, gpu_time_result);

    %% --- D. Sum the Phases for the Final Total ---
    % Total time is the sum of the time taken for each sequential phase.
    total_time = time_init + time_main + time_result;

    % --- E. Determine Bottleneck Status (Detailed HW Check with Needed CPUs/GPUs) ---
    is_cpu_hw_limited = false; % Flag for CPU HW limit
    is_gpu_hw_limited = false; % Flag for GPU HW limit
    is_cpu_sw_limited = false; % Separate flag for CPU SW limit
    is_gpu_sw_limited = false; % Separate flag for GPU SW limit
    
    needed_cpu_cores = 0; % Track maximum extra cores needed
    needed_gpu_cores = 0; % Track maximum extra cores needed

    % Check CPU phases for bottlenecks
    if SD_cores_cpu_init > total_cpu_cores
        is_cpu_hw_limited = true; 
        needed_cpu_cores = max(needed_cpu_cores, SD_cores_cpu_init - total_cpu_cores);
    elseif SD_cores_cpu_init > 0 && total_cpu_cores > 0
        is_cpu_sw_limited = true; 
    end
    if SD_cores_cpu_main > total_cpu_cores
        is_cpu_hw_limited = true; 
        needed_cpu_cores = max(needed_cpu_cores, SD_cores_cpu_main - total_cpu_cores);
    elseif SD_cores_cpu_main > 0 && total_cpu_cores > 0
        is_cpu_sw_limited = true; 
    end
     if SD_cores_cpu_result > total_cpu_cores
        is_cpu_hw_limited = true; 
        needed_cpu_cores = max(needed_cpu_cores, SD_cores_cpu_result - total_cpu_cores);
    elseif SD_cores_cpu_result > 0 && total_cpu_cores > 0
        is_cpu_sw_limited = true; 
    end

    % Check GPU phases for bottlenecks
    if SD_cores_gpu_init > total_gpu_cores
        is_gpu_hw_limited = true; 
        needed_gpu_cores = max(needed_gpu_cores, SD_cores_gpu_init - total_gpu_cores);
    elseif SD_cores_gpu_init > 0 && total_gpu_cores > 0
        is_gpu_sw_limited = true; 
    end
    if SD_cores_gpu_main > total_gpu_cores
        is_gpu_hw_limited = true; 
        needed_gpu_cores = max(needed_gpu_cores, SD_cores_gpu_main - total_gpu_cores);
    elseif SD_cores_gpu_main > 0 && total_gpu_cores > 0
        is_gpu_sw_limited = true; 
    end
    if SD_cores_gpu_result > total_gpu_cores
        is_gpu_hw_limited = true; 
        needed_gpu_cores = max(needed_gpu_cores, SD_cores_gpu_result - total_gpu_cores);
    elseif SD_cores_gpu_result > 0 && total_gpu_cores > 0
        is_gpu_sw_limited = true; 
    end

    % --- Calculate needed CPUs/GPUs ---
    needed_cpus = 0;
    if is_cpu_hw_limited && single_cpu_cores > 0
        needed_cpus = ceil(needed_cpu_cores / single_cpu_cores);
    end
    needed_gpus = 0;
    if is_gpu_hw_limited && single_gpu_cores > 0
        needed_gpus = ceil(needed_gpu_cores / single_gpu_cores);
    end
    
    % Final Bottleneck Summary (Detailed HW with Needed CPUs/GPUs)
    final_status = ''; % Initialize as char array
    if is_cpu_hw_limited && is_gpu_hw_limited
        % Use double for sprintf %f, then cast to int for %d
        final_status = sprintf('%d CPU(s) & %d GPU(s) needed - HW Limited', int32(needed_cpus), int32(needed_gpus));
    elseif is_cpu_hw_limited
        final_status = sprintf('%d more CPU(s) needed - HW Limited', int32(needed_cpus));
    elseif is_gpu_hw_limited
        final_status = sprintf('%d more GPU(s) needed - HW Limited', int32(needed_gpus));
    else
        % Check for SW limits only if not HW limited
        if is_cpu_sw_limited && is_gpu_sw_limited
            final_status = 'CPU & GPU SOFTWARE Limited';
        elseif is_cpu_sw_limited
            final_status = 'CPU SOFTWARE Limited';
        elseif is_gpu_sw_limited
            final_status = 'GPU SOFTWARE Limited';
        else
            final_status = 'Idle/Balanced'; % No significant bottlenecks
        end
    end

    % --- F. Assign the final status_text here ---
    % Explicitly convert the char array from sprintf to a string using string().
    status_text = string(final_status);
end
